simulink model "spring_dumper"  (Simulink 7.9)
settings: Solver=ode45  StartTime=0.0  StopTime=100  RelTol=1e-3
values from neighbouring files (symbols this model uses):
  c = 0.5    [spring_dumper_initial.m]
  k = 2    [spring_dumper_initial.m]
  m = 1    [spring_dumper_initial.m]
settings Model: Creator=Nice  LastModifiedBy=Nice

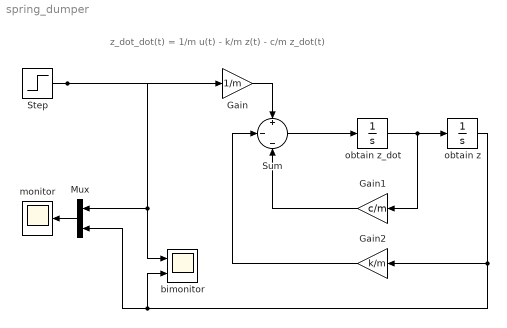
== system spring_dumper ==
  note: z_dot_dot(t) = 1/m u(t) - k/m z(t) - c/m z_dot(t)
  Gain : Gain  Gain=1/m
  Gain1 : Gain  Gain=c/m
  Gain2 : Gain  Gain=k/m
  Mux : Mux  Inputs=2
  Step : Step  SampleTime=0
  Sum : Sum  Inputs=+|-|-
  bimonitor : Scope  NumInputPorts=2
      settings: YMin=-5~-5  YMax=5~5
  monitor : Scope
  obtain z : Integrator
  obtain z_dot : Integrator
  wires:
  obtain z_dot/1 -> obtain z/1, Gain1/1
  obtain z/1 -> Gain2/1, bimonitor/2, Mux/2
  Step/1 -> Gain/1, bimonitor/1, Mux/1
  Gain/1 -> Sum/1
  Gain2/1 -> Sum/2
  Gain1/1 -> Sum/3
  Sum/1 -> obtain z_dot/1
  Mux/1 -> monitor/1
